simulink model "matlabfcn_whistlecount"  (R2017b)
settings: Solver=FixedStepAuto  StartTime=0.0  StopTime=inf  RelTol=1e-3
PreLoadFcn:
  | clear;
  | fs = 44100;
  | block_size = 0.5; %[sec]
  | block_size_samples = block_size*fs; % in samples
  | 
  | win = 0.05; % [sec] (frame size)
  | hop = 0.5*win;  % [sec] (hop size)
  | 
  | windowLength = round(win*fs);
  | hopSize = round(hop * fs);
  | load('SVMModel');
undefined symbols (not defined in the file): fdesignblkfcn, gcbh, mean_overallX, std_overallX
libraries: androidlib x3, dsparch4 x1, dspswit3 x1
settings Model: Creator=parva  LastModifiedBy=parva
settings OptimizationCC: PassReuseOutputArgsThreshold=0  MaxStackSize=64
settings DebuggingCC: ParameterTunabilityLossMsg=error
settings HardwareCC: ProdBitPerPointer=32  ProdBitPerSizeT=32  ProdBitPerPtrDiffT=32  ProdLargestAtomicInteger=Long  ProdLargestAtomicFloat=Double  ProdWordSize=32  ProdHWDeviceType=ARM Compatible->ARM Cortex  UseEmbeddedCoderFeatures=off
settings SFSimCC: MATLABDynamicMemAlloc=off
settings RTWCC: SystemTargetFile=ert.tlc  HardwareBoard=Android Device  TemplateMakefile=ert_default_tmf  GenerateReport=on  Toolchain=Android SDK/NDK Tools  LaunchReport=on
settings CodeAppCC: ForceParamTrailComments=on  OperatorAnnotations=on
settings ERTTargetCC: ERTCustomFileBanners=off  SupportContinuousTime=on  SupportNonInlinedSFcns=on  RemoveResetFunc=off  ModelStepFunctionPrototypeControlCompliant=off

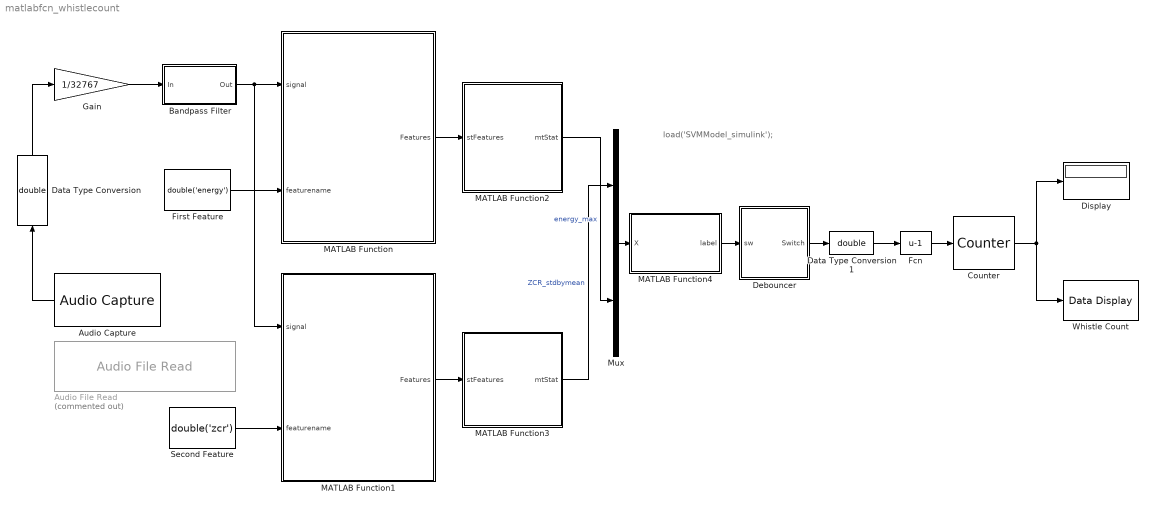
== system matlabfcn_whistlecount ==
  note: load('SVMModel_simulink');
  Audio Capture : androidlib/Audio Capture  SampleFreq=44100  FrameSize=22050  SampleTime=0.5  SimulateUsing=Code generation  DeviceStr=0  QueueDuration=0  BlockPlatform=Android  AudioSamplingFreq=44100
      settings: SourceProductName=Simulink Support Package for Android Devices  SourceProductBaseCode=ANDROID
  Audio File Read : androidlib/Audio File Read  Commented=on  FileName=C:\Users\parva\OneDrive\Documents\MATLAB\PressureCookerWhistleDetect\trial_svm\Test_data_and_code\distance_test_of_recordings\29122017_Koduvayur_rice_2metres.wav  FrameSize=block_size_samples
      settings: SourceProductName=Simulink Support Package for Android Devices  SourceProductBaseCode=ANDROID
  Bandpass Filter : Subsystem  DialogController=fdesignblkfcn  InitFcn=fdesignblkfcn(gcbh, {'InitFcn'});  mask(Bandpass Filter){}
      mask help: Design a bandpass filter
      settings: CopyFcn=fdesignblkfcn(gcbh, {'CopyFcn'});
      mask Help: helpview(mapfilelocation('dsp'), 'dspbandpassfilter');
      mask Display: disp('Bandpass');
  Counter : dspswit3/Counter  Direction=Up  CountEvent=Rising edge  CounterSize=User defined  MaxCount=255  InitialCount=0  Output=Count  HitValue=32  ResetInput=off  SamplesPerFrame=1  Ts=1  CntDtype=uint16  HitDtype=Logical
  Data Type Conversion : DataTypeConversion  OutDataTypeStr=double
  Data Type Conversion1 : DataTypeConversion  OutDataTypeStr=double
  Debouncer : Stateflow chart  TreatAsAtomicUnit=on
  Display : Display
  Fcn : Fcn  Expr=u-1
  First Feature : Constant  Value=double('energy')
  Gain : Gain  Gain=1/32767
  MATLAB Function : MATLAB Function  TreatAsAtomicUnit=on
  MATLAB Function1 : MATLAB Function  TreatAsAtomicUnit=on
  MATLAB Function2 : MATLAB Function  TreatAsAtomicUnit=on
  MATLAB Function3 : MATLAB Function  TreatAsAtomicUnit=on
  MATLAB Function4 : MATLAB Function  TreatAsAtomicUnit=on
  Mux : Mux  Inputs=2
  Second Feature : Constant  Value=double('zcr')
  Whistle Count : androidlib/Data Display  DataDisplayId=matlabfcn_whistlecount/Whistle_Count  Format=Integer  Precision=6  SimulateUsing=Code generation  blockPlatform=Android
      settings: SourceProductName=Simulink Support Package for Android Devices  SourceProductBaseCode=ANDROID
  wires:
  MATLAB Function4/1(label) -> Debouncer/1(sw)
  MATLAB Function1/1(Features) -> MATLAB Function3/1(stFeatures)
  Counter/1 -> Display/1, Whistle Count/1
  MATLAB Function2/1(mtStat) -> Mux/2  "energy_max"
  Data Type Conversion1/1 -> Fcn/1
  Fcn/1 -> Counter/1
  MATLAB Function3/1(mtStat) -> Mux/1  "ZCR_stdbymean"
  Bandpass Filter/1(Out) -> MATLAB Function/1(signal), MATLAB Function1/1(signal)
  Mux/1 -> MATLAB Function4/1(X)
  Debouncer/1(Switch) -> Data Type Conversion1/1
  First Feature/1 -> MATLAB Function/2(featurename)
  Second Feature/1 -> MATLAB Function1/2(featurename)
  Gain/1 -> Bandpass Filter/1(In)
  MATLAB Function/1(Features) -> MATLAB Function2/1(stFeatures)
  Data Type Conversion/1 -> Gain/1
  Audio Capture/1 -> Data Type Conversion/1

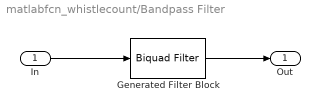
== system matlabfcn_whistlecount/Bandpass Filter ==
  In : Inport
  Generated Filter Block : dsparch4/Biquad Filter  Tag=BlockMethodSubSystem  IIRFiltStruct=Direct form II  CoeffSource=Specify via dialog  BiQuadCoeffs=[0.0255997931654626115 0 -0.0255997931654626115 1 -1.83957926135227701 0.982042265563317973;0.132513235910107025 0 -0.132513235910107025 1 -1.81598664651016684 0.975909375050803773;0.0752683347298045008 0 -0.0752683347298045008 1 -1.72689572035290029 0.970631606183356199;0.0225260226379304408 0 -0.0225260226379304408 1 -1.75710591593194732 0.969335715909204199;0.268270341371694643 0 -0.268270341371694643 1 -1.87037926991344605 0.996294571667002082;0.136007789782083083 0 -0.136007789782083083 1 -1.6805637273723788 0.994297939377325579;0.0431626037184006522 0 -0.0431626037184006522 1 -1.70134763803898936 0.975562130223233015;0.0293633766712807533 0 -0.0293633766712807533 1 -1.7878564576760505 0.971361196867287391;0.247656294233076696 0 -0.247656294233076696 1 -1.85778234932936193 0.988993537927781663;1.42641993216284435 0 -1.42641993216284435 1 -1.68476739265773023 0.983774381225085093]  a0Flag=Warning  IC=0  ICnum=0  ICden=0  InputProcessing=Columns as channels (frame based)  denAccumFracLength=30  denProdOutputFracLength=30  secondMemoryFracLength=15  roundingMode=Floor  overflowMode=off  ScaleValues=[0.00668361882128671973;1;1;1;1;1;1;1;1;1;1]  optimizeScaleValues=off  ScaleValueMode=Specify via input port (g)  scaleValueFracLength=14  FilterSource=Specify via dialog  FilterObject=BQF
      settings: SourceProductName=DSP System Toolbox
  Out : Outport
  wires:
  In/1 -> Generated Filter Block/1
  Generated Filter Block/1 -> Out/1

== matlab function matlabfcn_whistlecount/MATLAB Function1 ==
  data: Features output double; signal input; featurename input; windowLength parameter; hopSize parameter
function Features = st_Reduced_FeatureExtractBlock(signal, featurename, windowLength, hopSize)

featurename = convertCharsToStrings(char(featurename));
% % if STEREO ...
% if (size(signal,2)>1)
%     signal = (sum(signal,2)/2); % convert to MONO
% end
signal = (sum(signal,2)/2);
curPos = 1;
% L = block_size_samples;

% compute the total number of frames:
% numOfFrames = floor((L-windowLength)/hopSize) + 1;
numOfFrames = 18;

% number of features to be computed:
numOfFeatures = 1;
Features = zeros(numOfFeatures, numOfFrames);
% Ham = window(@hamming, windowLength);
Ham_vector = hamming(2205);
% frame = zeros(size(Ham_vector));
for i=1:numOfFrames % for each frame
    % get current frame:
    frame_orig  = signal(curPos:curPos+windowLength-1);
    frame = frame_orig.*Ham_vector;
%     for k = 1:length(Ham_vector)
%         frame(k)  = frame_orig(k)*Ham_vector(k);
%     end
    if (sum(abs(frame))>eps)
        % compute time-domain features:
        switch featurename
            case 'zcr'
                Features(1,i) = feature_zcr(frame);
            case 'energy'
                Features(1,i) = feature_energy(frame);
        end
    else
        Features(:,i) = zeros(numOfFeatures, 1);
    end
    curPos = curPos + hopSize;
end

== matlab function matlabfcn_whistlecount/MATLAB Function ==
  data: Features output double; signal input; featurename input; windowLength parameter; hopSize parameter
function Features = st_Reduced_FeatureExtractBlock(signal, featurename, windowLength, hopSize)

featurename = convertCharsToStrings(char(featurename));
% % if STEREO ...
% if (size(signal,2)>1)
%     signal = (sum(signal,2)/2); % convert to MONO
% end
signal = (sum(signal,2)/2);
curPos = 1;
% L = block_size_samples;

% compute the total number of frames:
% numOfFrames = floor((L-windowLength)/hopSize) + 1;
numOfFrames = 18;

% number of features to be computed:
numOfFeatures = 1;
Features = zeros(numOfFeatures, numOfFrames);
% Ham = window(@hamming, windowLength);
Ham_vector = hamming(2205);
% frame = zeros(size(Ham_vector));
for i=1:numOfFrames % for each frame
    % get current frame:
    frame_orig  = signal(curPos:curPos+windowLength-1);
    frame = frame_orig.*Ham_vector;
%     for k = 1:length(Ham_vector)
%         frame(k)  = frame_orig(k)*Ham_vector(k);
%     end
    if (sum(abs(frame))>eps)
        % compute time-domain features:
        switch featurename
            case 'zcr'
                Features(1,i) = feature_zcr(frame);
            case 'energy'
                Features(1,i) = feature_energy(frame);
        end
    else
        Features(:,i) = zeros(numOfFeatures, 1);
    end
    curPos = curPos + hopSize;
end

== matlab function matlabfcn_whistlecount/MATLAB Function2 ==
  data: stFeatures input; mtStat output
function mtStat  = mtStats_max(stFeatures)

[numOfFeatures, numOfStWins] = size(stFeatures);

curPos = 1;

mtWin = size(stFeatures,2);
mtStep = mtWin;

% compute the total number of mid-term frames:
numOfMidFrames = ceil((numOfStWins)/mtStep);
mtStat = zeros(numOfFeatures, numOfMidFrames);
% if (nargout==2)
%     shortFeaturesCell = cell(1, numOfMidFrames);
% end
for i=1:numOfMidFrames % for each mid-term frame
    % get current frame:
    N1 = curPos;
    N2 = curPos+mtWin-1;
    if (N2>size(stFeatures,2))
        N2 = size(stFeatures,2);
    end
    
    CurStFeatures  = stFeatures(:, N1:N2);
    
    %     for j=1:length(statistic)
    mtStat(:,i) = max(CurStFeatures');
    %     end
    curPos = curPos + mtStep;
end

% if strcmpi(statistic, 'stdbymean')
%     S = std(seq) ./ (mean(seq)+eps); return;
% end
% if strcmpi(statistic, 'max')
%     S = max(seq); return;
% end

== matlab function matlabfcn_whistlecount/MATLAB Function3 ==
  data: stFeatures input; mtStat output
function mtStat  = mtStats_stdbymean(stFeatures)

[numOfFeatures, numOfStWins] = size(stFeatures);

curPos = 1;

mtWin = size(stFeatures,2);
mtStep = mtWin;

% compute the total number of mid-term frames:
numOfMidFrames = ceil((numOfStWins)/mtStep);
mtStat = zeros(numOfFeatures, numOfMidFrames);

for i=1:numOfMidFrames % for each mid-term frame
    % get current frame:
    N1 = curPos;
    N2 = curPos+mtWin-1;
    if (N2>size(stFeatures,2))
        N2 = size(stFeatures,2);
    end
    
    CurStFeatures  = stFeatures(:, N1:N2);
    
    mtStat(:,i) = std(CurStFeatures') ./ (mean(CurStFeatures')+eps);
    
    curPos = curPos + mtStep;
end

% if strcmpi(statistic, 'stdbymean')
%     S = std(seq) ./ (mean(seq)+eps); return;
% end
% if strcmpi(statistic, 'max')
%     S = max(seq); return;
% end

== matlab function matlabfcn_whistlecount/MATLAB Function4 ==
  data: label output; X input; mean_overallX parameter; std_overallX parameter
function label = whistle_predict_fcn(X,mean_overallX,std_overallX) %#codegen
Mdl = loadCompactModel('SVMModel_simulink');

normalised_X = (X - mean_overallX')./std_overallX';
normalised_X_with_bias = [normalised_X',1];
label = predict(Mdl,normalised_X_with_bias);

end

== stateflow chart matlabfcn_whistlecount/Debouncer ==
  settings: updateMethod=DISCRETE  sampleTime=0.001
  state Off
  state On
  (default) -> Off
  On -> Off : [duration(sw <= 0) > 2]
  Off -> On : [duration(sw >= 1) >= 2]
  data: sw input; Switch output Enum: SwitchType
